simulink model "exp8_7"  (R2023a)
settings: Solver=VariableStepAuto  StartTime=0.0  StopTime=10.0  RelTol=1e-3
libraries: dspfdesign x1
settings Model: Creator=Lenovo  LastModifiedBy=Lenovo

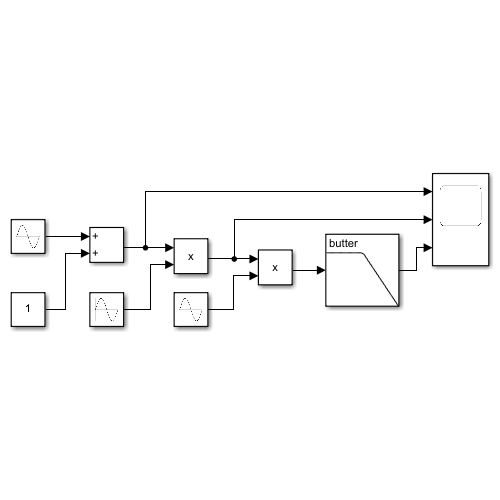
[thumbnail: Simulink's stored preview of the top-level diagram]
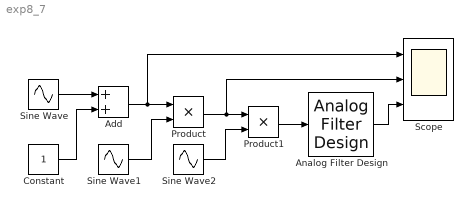
== system exp8_7 ==
  Add : Sum
  Analog Filter Design : dspfdesign/Analog Filter Design  method=Butterworth  filttype=Lowpass  N=8  Wlo=5  Whi=80  Rp=2  Rs=40
  Constant : Constant
  Product : Product
  Product1 : Product
  Scope : Scope  NumInputPorts=3
  Sine Wave : Sin  Frequency=5  SampleTime=0
  Sine Wave1 : Sin  Frequency=20  SampleTime=0
  Sine Wave2 : Sin  Frequency=20  SampleTime=0
  wires:
  Sine Wave/1 -> Add/1
  Constant/1 -> Add/2
  Sine Wave1/1 -> Product/2
  Product/1 -> Scope/2, Product1/1
  Sine Wave2/1 -> Product1/2
  Product1/1 -> Analog Filter Design/1
  Analog Filter Design/1 -> Scope/3
  Add/1 -> Scope/1, Product/1
